simulink model "ex5s"  (R2013a)
settings: Solver=ode45  StartTime=0.0  StopTime=10.0  RelTol=1e-3
undefined symbols (not defined in the file or in its folder): A, B, C, D
settings Model: Creator=Edward  LastModifiedBy=Edward

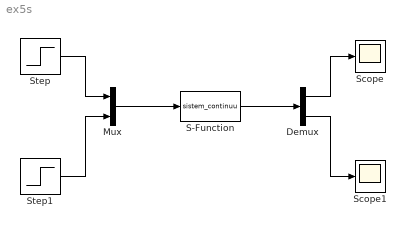
== system ex5s ==
  Demux : Demux  Outputs=2
  Mux : Mux  Inputs=2
  S-Function : S-Function  FunctionName=sistem_continuu  Parameters=A,B,C,D  EnableBusSupport=off
  Scope : Scope
  Scope1 : Scope
  Step : Step  SampleTime=0  ZeroCross=off
  Step1 : Step  SampleTime=0  ZeroCross=off
  wires:
  Mux/1 -> S-Function/1
  Step/1 -> Mux/1
  Step1/1 -> Mux/2
  S-Function/1 -> Demux/1
  Demux/1 -> Scope/1
  Demux/2 -> Scope1/1
